simulink model "chap05_01_15"  (R2013b)
settings: Solver=ode4  StartTime=5  StopTime=10  FixedStep=0.1  RelTol=1e-3
settings Model: Creator=Administrator  LastModifiedBy=sunzx.fnst
settings DataIOCC: InitialState=xFinal  LimitDataPoints=off  SaveOutput=off  SaveTime=off  ReturnWorkspaceOutputs=on
settings DebuggingCC: AlgebraicLoopMsg=error

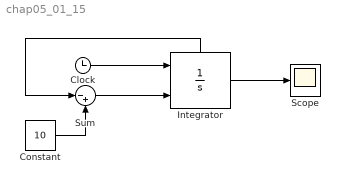
== system chap05_01_15 ==
  Clock : Clock
  Constant : Constant  Value=10
  Integrator : Integrator  ExternalReset=falling  ShowStatePort=on
  Scope : Scope
  Sum : Sum  Inputs=|-+
  wires:
  Clock/1 -> Integrator/1
  Constant/1 -> Sum/2
  Sum/1 -> Integrator/2
  Integrator/State -> Sum/1
  Integrator/1 -> Scope/1
